simulink library "CouplingSystemsLib"  (R2019b)
settings: Solver=VariableStepAuto  StartTime=0.0  StopTime=10.0  RelTol=1e-3
libraries: simulink x1
settings Model: ModifiedComment=mondt -- Thu May 26 19:01:11 2022 -- Version 1.12  Creator=cdyer  LastModifiedBy=ext-nadpurob
settings Model: ModifiedHistory=|
  | cdyer -- Mon Jan 22 16:33:05 2018 -- Version 1.11
  | - Upgrading to 2017b
settings DataIOCC: ReturnWorkspaceOutputs=off
settings DebuggingCC: ArithmeticOperatorsInVariantConditions=warning
settings SFSimCC: SimUseLocalCustomCode=off  CustomCodeUndefinedFunction=UseInterfaceOnly
settings RTWCC: RTWUseLocalCustomCode=off
settings CodeAppCC: StateflowObjectComments=on

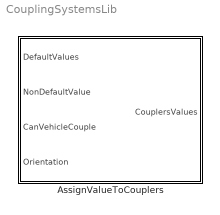
== system CouplingSystemsLib ==
  AssignValueToCouplers : Subsystem

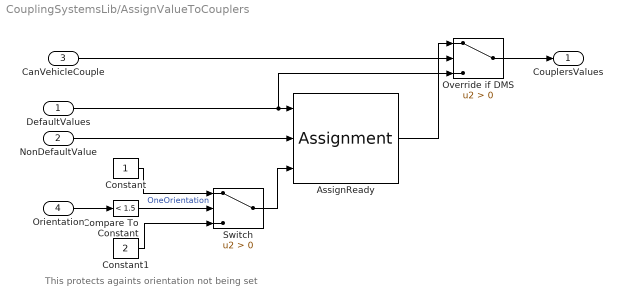
== system CouplingSystemsLib/AssignValueToCouplers ==
  note: This protects againts orientation not being set
  DefaultValues : Inport
  NonDefaultValue : Inport  Port=2
  CanVehicleCouple : Inport  Port=3
  Orientation : Inport  Port=4
  AssignReady : Assignment  DiagnosticForDimensions=Warning  IndexOptions=Index vector (port)  Indices=1  OutputSizes=1
  Compare To Constant : simulink/Logic and Bit Operations/Compare To Constant  relop=<  const=1.5  OutDataTypeStr=boolean
  Constant : Constant
  Constant1 : Constant  Value=2
  Override if DMS : Switch  Criteria=u2 > Threshold
  Switch : Switch  Criteria=u2 > Threshold
  CouplersValues : Outport  VectorParamsAs1DForOutWhenUnconnected=off
  wires:
  NonDefaultValue/1 -> AssignReady/2
  DefaultValues/1 -> AssignReady/1, Override if DMS/3
  AssignReady/1 -> Override if DMS/1
  Override if DMS/1 -> CouplersValues/1
  CanVehicleCouple/1 -> Override if DMS/2
  Orientation/1 -> Compare To Constant/1
  Switch/1 -> AssignReady/3
  Constant/1 -> Switch/1
  Constant1/1 -> Switch/3
  Compare To Constant/1 -> Switch/2  "OneOrientation"
